simulink model "EEBL_Scenario_01_cs"  (Simulink 7.6)
settings: Solver=ode5  SolverMode=SingleTasking  StartTime=0.0  StopTime=inf  FixedStep=1/100  RelTol=1e-3
PreLoadFcn:
  | check_NUTS_defined;
  | 
  | assignin('base',['model_closed_' bdroot],false);addpath('../includes_V2x');
InitFcn:
  | PreScanExperimentInitFcn(bdroot)
StopFcn:
  | PreScanExperimentStopFcn(bdroot)
undefined symbols (not defined in the file or in its folder): acceleration, actorID, actorType, DiscIntNeverNeededParam, GPS_alt, GPS_lat, GPS_long, intmax, lightBarInUse, messageID, publicVehicleType, rotZ, sireneInUse, trafficLightPriority, turnAdvice, velocity, x_ini_VRML, y_ini_VRML, yawRate, z_ini_VRML
libraries: simulink x58, PreScanSimulinkLibrary x12, simulink_extras x10, PreScanUsefulBlocks x6, simulink_need_slupdate x1
(part 10 of 10)

== system EEBL_Scenario_01_cs/Audi_A8_1/Dynamics_Simple/Chassis/MuxDynState/Transformation_BODY2GLOBAL ==
  Vvector_BODY_[m/s] : Inport
  angles_BODYwrtGLOB_[rad] : Inport  Port=2
  Dot Product : DotProduct  InputSameDT=on  OutDataTypeStr=Inherit: Inherit via internal rule
  Dot Product1 : DotProduct  InputSameDT=on  OutDataTypeStr=Inherit: Inherit via internal rule
  Dot Product2 : DotProduct  InputSameDT=on  OutDataTypeStr=Inherit: Inherit via internal rule
  Fcn10 : Fcn  Expr=cos(u(1))*sin(u(2))*sin(u(3))-sin(u(1))*cos(u(3))
  Fcn11 : Fcn  Expr=cos(u(1))*sin(u(2))*cos(u(3))+sin(u(1))*sin(u(3))
  Fcn12 : Fcn  Expr=sin(u(1))*cos(u(2))
  Fcn13 : Fcn  Expr=sin(u(1))*sin(u(2))*sin(u(3))+cos(u(1))*cos(u(3))
  Fcn14 : Fcn  Expr=sin(u(1))*sin(u(2))*cos(u(3))-cos(u(1))*sin(u(3))
  Fcn15 : Fcn  Expr=-sin(u(2))
  Fcn16 : Fcn  Expr=cos(u(2))*sin(u(3))
  Fcn17 : Fcn  Expr=cos(u(2))*cos(u(3))
  Fcn9 : Fcn  Expr=cos(u(1))*cos(u(2))
  Mux1 : Mux  Inputs=9
  Mux3 : Mux  Inputs=3
  Selector : Selector  InputPortWidth=9  IndexOptions=Index vector (dialog)  Indices=[1 2 3]  OutputSizes=1
  Selector1 : Selector  InputPortWidth=9  IndexOptions=Index vector (dialog)  Indices=[4 5 6]  OutputSizes=1
  Selector2 : Selector  InputPortWidth=9  IndexOptions=Index vector (dialog)  Indices=[7 8 9]  OutputSizes=1
  rot_xyz 2 rot_zyx : Selector  InputPortWidth=3  IndexOptions=Index vector (dialog)  Indices=[3 2 1]  OutputSizes=1
  Vvector_GLOBAL_[m/s] : Outport
  wires:
  Fcn9/1 -> Mux1/1
  Fcn10/1 -> Mux1/2
  Fcn11/1 -> Mux1/3
  Fcn12/1 -> Mux1/4
  Fcn13/1 -> Mux1/5
  Fcn14/1 -> Mux1/6
  Fcn15/1 -> Mux1/7
  Fcn16/1 -> Mux1/8
  Fcn17/1 -> Mux1/9
  Mux1/1 -> Selector/1, Selector1/1, Selector2/1  "RotationMatrix Visu"
  Selector/1 -> Dot Product/2
  Vvector_BODY_[m/s]/1 -> Dot Product2/1, Dot Product1/1, Dot Product/1
  Dot Product/1 -> Mux3/1
  Selector1/1 -> Dot Product1/2
  Selector2/1 -> Dot Product2/2
  Dot Product2/1 -> Mux3/3
  Dot Product1/1 -> Mux3/2
  rot_xyz 2 rot_zyx/1 -> Fcn9/1, Fcn10/1, Fcn11/1, Fcn12/1, Fcn13/1, Fcn14/1, Fcn15/1, Fcn16/1, Fcn17/1
  Mux3/1 -> Vvector_GLOBAL_[m/s]/1
  angles_BODYwrtGLOB_[rad]/1 -> rot_xyz 2 rot_zyx/1

== system EEBL_Scenario_01_cs/Audi_A8_1/Dynamics_Simple/Chassis/RearTyre/AlphaRear ==
  In : Inport
  Abs : Abs
  Compare To Constant : simulink/Logic and Bit Operations/Compare To Constant  SystemSampleTime=-1  relop=>  const=0  LogicOutDataTypeMode=uint8  ZeroCross=off
  Enabled Subsystem : Subsystem  TreatAsAtomicUnit=on
  Selector : Selector  IndexOptions=Index vector (dialog)  Indices=1  OutputSizes=1
  Alpha : Outport
  wires:
  Selector/1 -> Abs/1
  Compare To Constant/1 -> Enabled Subsystem/Enable
  Enabled Subsystem/1(Alpha) -> Alpha/1
  In/1 -> Enabled Subsystem/1(In), Selector/1
  Abs/1 -> Compare To Constant/1

== system EEBL_Scenario_01_cs/Audi_A8_1/Dynamics_Simple/Chassis/RearTyre/Configurable Subsystem ==
  In1 : Inport
  In2 : Inport  Port=2
  Integrator : Integrator  ExternalReset=level
  Out1 : Outport
  wires:
  In1/1 -> Integrator/1
  In2/1 -> Integrator/2
  Integrator/1 -> Out1/1

== system EEBL_Scenario_01_cs/Audi_A8_1/Dynamics_Simple/Chassis/RearTyre/Configurable Subsystem1 ==
  In1 : Inport
  In2 : Inport  Port=2
  Integrator : Integrator  ExternalReset=level  LimitOutput=on  UpperSaturationLimit=1  LowerSaturationLimit=-1
  Out1 : Outport
  wires:
  In1/1 -> Integrator/1
  In2/1 -> Integrator/2
  Integrator/1 -> Out1/1

== system EEBL_Scenario_01_cs/Audi_A8_1/Dynamics_Simple/ShiftLogic/Detect Increase/If V0 higher of the from 2->3 shifting velocity ==
  In1 : Inport
  Action Port : ActionPort  PropagateVarSize=During execution  ActionType=then
  Out1 : Outport
  wires:
  In1/1 -> Out1/1

== system EEBL_Scenario_01_cs/Audi_A8_1/Dynamics_Simple/ShiftLogic/Detect Increase/Other ==
  In1 : Inport
  Action Port : ActionPort  PropagateVarSize=During execution  ActionType=else
  Data Type Conversion : DataTypeConversion  OutDataTypeStr=double
  Detect Increase : simulink/Logic and Bit Operations/Detect Increase  SystemSampleTime=-1  vinit=0.0
  Out1 : Outport
  wires:
  In1/1 -> Detect Increase/1
  Detect Increase/1 -> Data Type Conversion/1
  Data Type Conversion/1 -> Out1/1

== system EEBL_Scenario_01_cs/Audi_A8_1/Dynamics_Simple/Transmission/Transmission_Ratio/If Action Neutral ==
  In1 : Inport
  Action Port : ActionPort  InitializeStates=reset  PropagateVarSize=During execution  ActionType=then
  Out1 : Outport
  wires:
  In1/1 -> Out1/1

== system EEBL_Scenario_01_cs/Audi_A8_1/Dynamics_Simple/Transmission/Transmission_Ratio/If Action Normal ==
  In1 : Inport
  Action Port : ActionPort  InitializeStates=reset  PropagateVarSize=During execution  ActionType=else
  Out1 : Outport
  wires:
  In1/1 -> Out1/1

== system EEBL_Scenario_01_cs/Audi_A8_1/Dynamics_Simple/Transmission/Transmission_Ratio/If Action Reverse ==
  In1 : Inport
  Action Port : ActionPort  InitializeStates=reset  PropagateVarSize=During execution  ActionType=elseif
  Reverse : Gain  Gain=-1
  Out1 : Outport
  wires:
  Reverse/1 -> Out1/1
  In1/1 -> Reverse/1

== system EEBL_Scenario_01_cs/Audi_A8_1/Trajectories/Traj2State1/Traj2State2/MuxState ==
  x [m] : Inport
  y [m] : Inport  Port=2
  z [m] : Inport  Port=3
  dx [m/s] : Inport  Port=4
  dy [m/s] : Inport  Port=5
  dz [m/s] : Inport  Port=6
  R [rad] : Inport  Port=7
  P [rad] : Inport  Port=8
  Y [rad] : Inport  Port=9
  Mux : Mux  Inputs=9
  state : Outport
  wires:
  z [m]/1 -> Mux/3
  y [m]/1 -> Mux/2
  x [m]/1 -> Mux/1
  Y [rad]/1 -> Mux/9
  P [rad]/1 -> Mux/8
  R [rad]/1 -> Mux/7
  dz [m/s]/1 -> Mux/6
  dy [m/s]/1 -> Mux/5
  dx [m/s]/1 -> Mux/4
  Mux/1 -> state/1

== system EEBL_Scenario_01_cs/Audi_A8_1/Trajectories/Traj2State1/Traj2State2/Traj2MuxState_Ext ==
  Traj : Inport
  Terminator{1..9} (9 alike) : Terminator
  demux : Subsystem
  x [m] : Outport
  y [m] : Outport  Port=2
  z [m] : Outport  Port=3
  dx [m/s] : Outport  Port=4
  dy [m/s] : Outport  Port=5
  dz [m/s] : Outport  Port=6
  R [rad] : Outport  Port=7
  P [rad] : Outport  Port=8
  Y [rad] : Outport  Port=9
  wires:
  demux/9(Y) -> Y [rad]/1
  demux/7(R) -> R [rad]/1
  demux/5(vely) -> dy [m/s]/1
  demux/4(velx) -> dx [m/s]/1
  demux/10(velR) -> Terminator4/1
  demux/11(velP) -> Terminator5/1
  demux/12(velY) -> Terminator1/1
  demux/13(accx) -> Terminator8/1
  demux/14(accy) -> Terminator9/1
  demux/15(accz) -> Terminator7/1
  demux/18(accY) -> Terminator2/1
  demux/16(accR) -> Terminator3/1
  demux/17(accP) -> Terminator6/1
  demux/3(z) -> z [m]/1
  Traj/1 -> demux/1(traj)
  demux/6(velz) -> dz [m/s]/1
  demux/1(x) -> x [m]/1
  demux/2(y) -> y [m]/1
  demux/8(P) -> P [rad]/1

== system EEBL_Scenario_01_cs/BMW_X5_1/Trajectories/ElapsedTrack1/MuxState/Substitute 90 & 270 deg (and its plurals) ==
  Angle [rad] : Inport
  270 deg detection : simulink/Model Verification/Check  Static Gap  Description=u <= 269.5 || 270.5 <= u  SystemSampleTime=-1  max=270.5  max_included=on  min=269.5  min_included=on  enabled=on  stopWhenAssertionFail=off  export=on  icon=graphic
  90 deg detection : simulink/Model Verification/Check  Static Gap  Description=u <= 89.5 || 90.5 <= u  SystemSampleTime=-1  max=90.5  max_included=on  min=89.5  min_included=on  enabled=on  stopWhenAssertionFail=off  export=on  icon=graphic
  Angle 0-360 deg limiter : Subsystem
  Degrees to Radians : simulink_extras/Transformations/Degrees to Radians  SystemSampleTime=-1
  Radians to Degrees : simulink_extras/Transformations/Radians to Degrees  SystemSampleTime=-1
  Substitution  Value : Constant  Value=269.5
  Substitution Value : Constant  Value=89.5
  Switch : Switch  Threshold=0.5
  Switch1 : Switch  Threshold=0.5
  Subst Angle [rad] : Outport
  wires:
  Angle [rad]/1 -> Radians to Degrees/1
  Degrees to Radians/1 -> Subst Angle [rad]/1
  Radians to Degrees/1 -> Angle 0-360 deg limiter/1(Angle [deg])
  Switch1/1 -> Degrees to Radians/1
  Substitution  Value/1 -> Switch1/3
  270 deg detection/1 -> Switch1/2
  Switch/1 -> Switch1/1, 270 deg detection/1
  Substitution Value/1 -> Switch/3
  90 deg detection/1 -> Switch/2
  Angle 0-360 deg limiter/1(LimAngle [deg]) -> 90 deg detection/1, Switch/1

== system EEBL_Scenario_01_cs/BMW_X5_1/Trajectories/Traj2State1/Traj2State2/MuxState ==
  x [m] : Inport
  y [m] : Inport  Port=2
  z [m] : Inport  Port=3
  dx [m/s] : Inport  Port=4
  dy [m/s] : Inport  Port=5
  dz [m/s] : Inport  Port=6
  R [rad] : Inport  Port=7
  P [rad] : Inport  Port=8
  Y [rad] : Inport  Port=9
  Mux : Mux  Inputs=9
  state : Outport
  wires:
  z [m]/1 -> Mux/3
  y [m]/1 -> Mux/2
  x [m]/1 -> Mux/1
  Y [rad]/1 -> Mux/9
  P [rad]/1 -> Mux/8
  R [rad]/1 -> Mux/7
  dz [m/s]/1 -> Mux/6
  dy [m/s]/1 -> Mux/5
  dx [m/s]/1 -> Mux/4
  Mux/1 -> state/1

== system EEBL_Scenario_01_cs/BMW_X5_1/Trajectories/Traj2State1/Traj2State2/Traj2MuxState_Ext ==
  Traj : Inport
  Terminator{1..9} (9 alike) : Terminator
  demux : Subsystem
  x [m] : Outport
  y [m] : Outport  Port=2
  z [m] : Outport  Port=3
  dx [m/s] : Outport  Port=4
  dy [m/s] : Outport  Port=5
  dz [m/s] : Outport  Port=6
  R [rad] : Outport  Port=7
  P [rad] : Outport  Port=8
  Y [rad] : Outport  Port=9
  wires:
  demux/9(Y) -> Y [rad]/1
  demux/7(R) -> R [rad]/1
  demux/5(vely) -> dy [m/s]/1
  demux/4(velx) -> dx [m/s]/1
  demux/10(velR) -> Terminator4/1
  demux/11(velP) -> Terminator5/1
  demux/12(velY) -> Terminator1/1
  demux/13(accx) -> Terminator8/1
  demux/14(accy) -> Terminator9/1
  demux/15(accz) -> Terminator7/1
  demux/18(accY) -> Terminator2/1
  demux/16(accR) -> Terminator3/1
  demux/17(accP) -> Terminator6/1
  demux/3(z) -> z [m]/1
  Traj/1 -> demux/1(traj)
  demux/6(velz) -> dz [m/s]/1
  demux/1(x) -> x [m]/1
  demux/2(y) -> y [m]/1
  demux/8(P) -> P [rad]/1

== system EEBL_Scenario_01_cs/BMW_X5_1/vehicle CAM generator/CAM generation/maybe/If Action Subsystem ==
  x [m] : Inport
  y [m] : Inport  Port=2
  z [m] : Inport  Port=3
  rotZ [deg] : Inport  Port=4
  velocity [m/s] : Inport  Port=5
  Action Port : ActionPort  PropagateVarSize=During execution  ActionType=then
  Constant : Constant
  Data Store Write : DataStoreWrite  DataStoreName=CAM_velocity
  Data Store Write1 : DataStoreWrite  DataStoreName=CAM_heading
  Data Store Write2 : DataStoreWrite  DataStoreName=CAM_x
  Data Store Write3 : DataStoreWrite  DataStoreName=CAM_y
  Data Store Write4 : DataStoreWrite  DataStoreName=CAM_z
  Data Store Write5 : DataStoreWrite  DataStoreName=CAM_time
  Digital Clock1 : DigitalClock  SampleTime=0.01
  Out1 : Outport  InitialOutput=0
  wires:
  Constant/1 -> Out1/1
  velocity [m/s]/1 -> Data Store Write/1
  rotZ [deg]/1 -> Data Store Write1/1
  x [m]/1 -> Data Store Write2/1
  y [m]/1 -> Data Store Write3/1
  z [m]/1 -> Data Store Write4/1
  Digital Clock1/1 -> Data Store Write5/1

== system EEBL_Scenario_01_cs/BMW_X5_1/vehicle CAM generator/CAM generation/maybe/If Action Subsystem1 ==
  Action Port : ActionPort  PropagateVarSize=During execution  ActionType=else
  Constant : Constant  Value=0
  Out1 : Outport  InitialOutput=0
  wires:
  Constant/1 -> Out1/1

== system EEBL_Scenario_01_cs/Audi_A8_1/Dynamics_Simple/Chassis/Bicycle_model_[XYZ]/X_Motion/Air&RoadResistance ==
  vx_[ms-1] : Inport
  Gain : Gain  Gain=1/p.Rw
  Road & Aerodyn Resistances : Fcn  Expr=p.Rroad + p.Rair*u^2
  Saturation1 : Saturate  UpperLimit=5/15  LowerLimit=-5/15
  Sign : Signum
  "[ms-1] 2 [rads-1]" : Gain  Gain=1/p.Rw  SaturateOnIntegerOverflow=on  OutDataTypeStr=Inherit: Same as input  ParamDataTypeStr=Inherit: Same as input
  signed load1 : Product  SaturateOnIntegerOverflow=on  InputSameDT=on  OutDataTypeStr=Inherit: Same as first input
  Resistance_Force : Outport
  wires:
  signed load1/1 -> Resistance_Force/1  "F_[N]"
  vx_[ms-1]/1 -> Road & Aerodyn Resistances/1, "[ms-1] 2 [rads-1]"/1
  Saturation1/1 -> Sign/1
  "[ms-1] 2 [rads-1]"/1 -> Saturation1/1
  Road & Aerodyn Resistances/1 -> Gain/1  "ResistanceTorque_[Nm]"
  Sign/1 -> signed load1/2  "sign"
  Gain/1 -> signed load1/1  "Resistance Force_[N]"

== system EEBL_Scenario_01_cs/Audi_A8_1/Dynamics_Simple/Chassis/Bicycle_model_[XYZ]/X_Motion/BrakeSystem ==
  vx_[ms-1] : Inport
  BrakePressure_[bar] : Inport  Port=2
  Gain : Gain  Gain=1/p.Rw
  Saturation : Saturate  UpperLimit=p.PBrakeMax  LowerLimit=0
  Saturation1 : Saturate  UpperLimit=5/15  LowerLimit=-5/15
  Sign : Signum
  "[ms-1] 2 [rads-1]" : Gain  Gain=1/p.Rw  SaturateOnIntegerOverflow=on  OutDataTypeStr=Inherit: Same as input  ParamDataTypeStr=Inherit: Same as input
  braking Q factor : Gain  Gain=p.Qfac  SaturateOnIntegerOverflow=on  OutDataTypeStr=Inherit: Same as input  ParamDataTypeStr=Inherit: Same as input
  signed load1 : Product  SaturateOnIntegerOverflow=on  InputSameDT=on  OutDataTypeStr=Inherit: Same as first input
  BrakeForce : Outport
  BrakeTorqueAbs : Outport  Port=2
  wires:
  braking Q factor/1 -> BrakeTorqueAbs/1, Gain/1
  BrakePressure_[bar]/1 -> Saturation/1
  Saturation/1 -> braking Q factor/1
  vx_[ms-1]/1 -> "[ms-1] 2 [rads-1]"/1
  Saturation1/1 -> Sign/1
  "[ms-1] 2 [rads-1]"/1 -> Saturation1/1
  Sign/1 -> signed load1/2  "sign"
  signed load1/1 -> BrakeForce/1
  Gain/1 -> signed load1/1

== system EEBL_Scenario_01_cs/Audi_A8_1/Dynamics_Simple/Chassis/Bicycle_model_[XYZ]/X_Motion/Configurable Subsystem ==
  In1 : Inport
  In2 : Inport  Port=2
  In3 : Inport  Port=3
  Integrator : Integrator  ExternalReset=level  InitialConditionSource=external
  Out1 : Outport
  wires:
  In1/1 -> Integrator/1
  In2/1 -> Integrator/2
  In3/1 -> Integrator/3
  Integrator/1 -> Out1/1

== system EEBL_Scenario_01_cs/Audi_A8_1/Dynamics_Simple/Chassis/Bicycle_model_[XYZ]/X_Motion/Configurable Subsystem1 ==
  In1 : Inport
  Torsional damping : TransferFcn  Denominator=[0.1 1]
  Out1 : Outport
  wires:
  In1/1 -> Torsional damping/1
  Torsional damping/1 -> Out1/1

== system EEBL_Scenario_01_cs/Audi_A8_1/Dynamics_Simple/Chassis/Bicycle_model_[XYZ]/X_Motion/Max RPM and zero- velocity detection ==
  note: Set to zero after infinite small time-step
  note: Zero velocity detection
  ax : Inport
  Drive Torque : Inport  Port=2
  Brake Torque : Inport  Port=3
  v0 : Inport  Port=4
  vx : Inport  Port=5
  Abs : Abs
  Abs1 : Abs
  Compare To Zero : simulink/Logic and Bit Operations/Compare To Zero  SystemSampleTime=-1  relop=<=  LogicOutDataTypeMode=boolean  ZeroCross=off
  Compare To Zero1 : simulink/Logic and Bit Operations/Compare To Zero  SystemSampleTime=-1  relop=>=  LogicOutDataTypeMode=boolean  ZeroCross=off
  Compare To Zero2 : simulink/Logic and Bit Operations/Compare To Zero  SystemSampleTime=-1  relop=>=  LogicOutDataTypeMode=boolean  ZeroCross=off
  Compare To Zero3 : simulink/Logic and Bit Operations/Compare To Zero  SystemSampleTime=-1  relop=<=  LogicOutDataTypeMode=boolean  ZeroCross=off
  Configurable Subsystem : Subsystem  BlockChoice=Step  mask{ComputationMode=ComputationMode}
      mask prompts: ComputationMode "Compuation mode:"
      mask init:
      | SetComputationMode(gcb,ComputationMode);
      settings: AttributesFormatString=%<BlockChoice>  OpenFcn=BringToFront(gcb);  MemberBlocks=Discrete Step,Step
      settings: TemplateBlock=|
      | PreScanSimulinkLibrary/Configurable Subsystems/Step Function/Configurable
      | Subsystem
  Constant : Constant
  Constant1 : Constant
  Logical Operator : Logic  AllPortsSameDT=off  OutDataTypeStr=boolean
  Logical Operator1 : Logic  AllPortsSameDT=off  OutDataTypeStr=boolean
  Logical Operator2 : Logic  Operator=NOT  AllPortsSameDT=off  OutDataTypeStr=boolean
  Logical Operator3 : Logic  AllPortsSameDT=off  OutDataTypeStr=boolean
  Logical Operator4 : Logic  Operator=OR  AllPortsSameDT=off  OutDataTypeStr=boolean
  Memory : Memory
  Memory1 : Memory
  Memory2 : Memory
  Product : Product  RndMeth=Zero
  Relational Operator : RelationalOperator  Operator=<  OutDataTypeStr=boolean
  SR-Memory : Subsystem
  Sum : Sum  Inputs=|-+
  Switch : Switch  Criteria=u2 ~= 0  Threshold=0.5
  ax is 0 : Constant  Value=0
  ax_out : Outport
  vx_reset : Outport  Port=2
  x0 : Outport  Port=3
  wires:
  Logical Operator4/1 -> Logical Operator1/1
  vx/1 -> Compare To Zero/1, Compare To Zero2/1, Memory2/1, Memory/1  "vx"
  Memory2/1 -> Compare To Zero3/1
  Compare To Zero2/1 -> Logical Operator3/1
  Compare To Zero3/1 -> Logical Operator3/2
  Logical Operator3/1 -> Logical Operator4/2  "zero-crossing backward"
  Memory/1 -> Compare To Zero1/1
  Compare To Zero/1 -> Logical Operator/1
  Compare To Zero1/1 -> Logical Operator/2
  Logical Operator/1 -> Logical Operator4/1  "zero-crossing forward"
  Abs/1 -> Relational Operator/1
  Abs1/1 -> Relational Operator/2
  Drive Torque/1 -> Abs/1
  Brake Torque/1 -> Abs1/1
  Relational Operator/1 -> Logical Operator1/2, Logical Operator2/1
  Logical Operator1/1 -> SR-Memory/2(Set)
  Constant/1 -> SR-Memory/1(Signal)
  Logical Operator2/1 -> SR-Memory/3(Reset)
  SR-Memory/1(Out) -> Sum/1, Memory1/1
  Switch/1 -> ax_out/1
  Sum/1 -> Switch/2
  ax is 0/1 -> Switch/3
  Constant1/1 -> Sum/2
  v0/1 -> Product/1
  Product/1 -> x0/1
  Configurable Subsystem/1(Out1) -> Product/2
  ax/1 -> Switch/1  "ax"
  Memory1/1 -> vx_reset/1  "vx"

== system EEBL_Scenario_01_cs/Audi_A8_1/Dynamics_Simple/Chassis/Bicycle_model_[XYZ]/Y & Yaw_Motion/Configurable Subsystem ==
  In1 : Inport
  In2 : Inport  Port=2
  Integrator : Integrator  ExternalReset=level
  Out1 : Outport
  wires:
  In1/1 -> Integrator/1
  In2/1 -> Integrator/2
  Integrator/1 -> Out1/1

== system EEBL_Scenario_01_cs/Audi_A8_1/Dynamics_Simple/Chassis/Bicycle_model_[XYZ]/Y & Yaw_Motion/Configurable Subsystem1 ==
  In1 : Inport
  Integrator : Integrator
  Out1 : Outport
  wires:
  In1/1 -> Integrator/1
  Integrator/1 -> Out1/1

== system EEBL_Scenario_01_cs/Audi_A8_1/Dynamics_Simple/Chassis/Bicycle_model_[XYZ]/Y & Yaw_Motion/Configurable Subsystem2 ==
  In1 : Inport
  In2 : Inport  Port=2
  Integrator : Integrator  ExternalReset=level
  Out1 : Outport
  wires:
  In1/1 -> Integrator/1
  In2/1 -> Integrator/2
  Integrator/1 -> Out1/1

== system EEBL_Scenario_01_cs/Audi_A8_1/Dynamics_Simple/Chassis/Bicycle_model_[XYZ]/Z, Pitch_Motion & Roll_Motion/Configurable Subsystem ==
  In1 : Inport
  Integrator : Integrator  LimitOutput=on  UpperSaturationLimit=5*pi/180  LowerSaturationLimit=-5*pi/180
  Out1 : Outport
  wires:
  In1/1 -> Integrator/1
  Integrator/1 -> Out1/1

== system EEBL_Scenario_01_cs/Audi_A8_1/Dynamics_Simple/Chassis/Bicycle_model_[XYZ]/Z, Pitch_Motion & Roll_Motion/Configurable Subsystem1 ==
  In1 : Inport
  Integrator : Integrator
  Out1 : Outport
  wires:
  In1/1 -> Integrator/1
  Integrator/1 -> Out1/1

== system EEBL_Scenario_01_cs/Audi_A8_1/Dynamics_Simple/Chassis/Bicycle_model_[XYZ]/Z, Pitch_Motion & Roll_Motion/Configurable Subsystem2 ==
  In1 : Inport
  Integrator : Integrator
  Out1 : Outport
  wires:
  In1/1 -> Integrator/1
  Integrator/1 -> Out1/1

== system EEBL_Scenario_01_cs/Audi_A8_1/Dynamics_Simple/Chassis/Bicycle_model_[XYZ]/Z, Pitch_Motion & Roll_Motion/Configurable Subsystem3 ==
  In1 : Inport
  Integrator : Integrator
  Out1 : Outport
  wires:
  In1/1 -> Integrator/1
  Integrator/1 -> Out1/1

== system EEBL_Scenario_01_cs/Audi_A8_1/Dynamics_Simple/Chassis/Bicycle_model_[XYZ]/Z, Pitch_Motion & Roll_Motion/Configurable Subsystem4 ==
  In1 : Inport
  Integrator : Integrator
  Out1 : Outport
  wires:
  In1/1 -> Integrator/1
  Integrator/1 -> Out1/1

== system EEBL_Scenario_01_cs/Audi_A8_1/Dynamics_Simple/Chassis/Bicycle_model_[XYZ]/Z, Pitch_Motion & Roll_Motion/Configurable Subsystem5 ==
  In1 : Inport
  Integrator : Integrator
  Out1 : Outport
  wires:
  In1/1 -> Integrator/1
  Integrator/1 -> Out1/1

== system EEBL_Scenario_01_cs/Audi_A8_1/Dynamics_Simple/Chassis/Bicycle_model_[XYZ]/Z, Pitch_Motion & Roll_Motion/Configurable Subsystem9 ==
  In1 : Inport
  Derivative : Derivative
  Out1 : Outport
  wires:
  In1/1 -> Derivative/1
  Derivative/1 -> Out1/1

== system EEBL_Scenario_01_cs/Audi_A8_1/Dynamics_Simple/Chassis/FrontTyre/AlphaFront/Enabled Subsystem ==
  In : Inport
  Enable : EnablePort  PropagateVarSize=During execution
  AlphaFront : Fcn  Expr=-atan( (u(2)+u(3)*p.a)/u(1) )
  Alpha : Outport  OutputWhenDisabled=reset  InitialOutput=[0]
  wires:
  AlphaFront/1 -> Alpha/1
  In/1 -> AlphaFront/1

== system EEBL_Scenario_01_cs/Audi_A8_1/Dynamics_Simple/Chassis/RearTyre/AlphaRear/Enabled Subsystem ==
  In : Inport
  Enable : EnablePort  PropagateVarSize=During execution
  AlphaRear : Fcn  Expr=-atan( (u(2)-u(3)*p.b)/u(1) )
  Alpha : Outport  OutputWhenDisabled=reset  InitialOutput=[0]
  wires:
  AlphaRear/1 -> Alpha/1
  In/1 -> AlphaRear/1

== system EEBL_Scenario_01_cs/Audi_A8_1/Trajectories/Traj2State1/Traj2State2/Traj2MuxState_Ext/demux ==
  traj : Inport
  Demux : Demux  Outputs=18
  x : Outport
  y : Outport  Port=2
  z : Outport  Port=3
  velx : Outport  Port=4
  vely : Outport  Port=5
  velz : Outport  Port=6
  R : Outport  Port=7
  P : Outport  Port=8
  Y : Outport  Port=9
  velR : Outport  Port=10
  velP : Outport  Port=11
  velY : Outport  Port=12
  accx : Outport  Port=13
  accy : Outport  Port=14
  accz : Outport  Port=15
  accR : Outport  Port=16
  accP : Outport  Port=17
  accY : Outport  Port=18
  wires:
  Demux/18 -> accY/1
  Demux/17 -> accP/1
  Demux/16 -> accR/1
  Demux/15 -> accz/1
  Demux/14 -> accy/1
  Demux/13 -> accx/1
  Demux/12 -> velY/1
  Demux/11 -> velP/1
  Demux/10 -> velR/1
  Demux/9 -> velz/1
  Demux/8 -> vely/1
  Demux/7 -> velx/1
  Demux/6 -> Y/1
  Demux/5 -> P/1
  traj/1 -> Demux/1
  Demux/4 -> R/1
  Demux/3 -> z/1
  Demux/2 -> y/1
  Demux/1 -> x/1

== system EEBL_Scenario_01_cs/BMW_X5_1/Trajectories/ElapsedTrack1/MuxState/Substitute 90 & 270 deg (and its plurals)/Angle 0-360 deg limiter ==
  Angle [deg] : Inport
  Gain : Gain  Gain=1/360
  Gain1 : Gain  Gain=360
  Rounding Function : Rounding
  Sum : Sum  Inputs=|-+
  LimAngle [deg] : Outport
  wires:
  Gain/1 -> Rounding Function/1
  Rounding Function/1 -> Gain1/1
  Gain1/1 -> Sum/1
  Angle [deg]/1 -> Gain/1, Sum/2
  Sum/1 -> LimAngle [deg]/1

== system EEBL_Scenario_01_cs/BMW_X5_1/Trajectories/Traj2State1/Traj2State2/Traj2MuxState_Ext/demux ==
  traj : Inport
  Demux : Demux  Outputs=18
  x : Outport
  y : Outport  Port=2
  z : Outport  Port=3
  velx : Outport  Port=4
  vely : Outport  Port=5
  velz : Outport  Port=6
  R : Outport  Port=7
  P : Outport  Port=8
  Y : Outport  Port=9
  velR : Outport  Port=10
  velP : Outport  Port=11
  velY : Outport  Port=12
  accx : Outport  Port=13
  accy : Outport  Port=14
  accz : Outport  Port=15
  accR : Outport  Port=16
  accP : Outport  Port=17
  accY : Outport  Port=18
  wires:
  Demux/18 -> accY/1
  Demux/17 -> accP/1
  Demux/16 -> accR/1
  Demux/15 -> accz/1
  Demux/14 -> accy/1
  Demux/13 -> accx/1
  Demux/12 -> velY/1
  Demux/11 -> velP/1
  Demux/10 -> velR/1
  Demux/9 -> velz/1
  Demux/8 -> vely/1
  Demux/7 -> velx/1
  Demux/6 -> Y/1
  Demux/5 -> P/1
  traj/1 -> Demux/1
  Demux/4 -> R/1
  Demux/3 -> z/1
  Demux/2 -> y/1
  Demux/1 -> x/1

== system EEBL_Scenario_01_cs/Audi_A8_1/Dynamics_Simple/Chassis/Bicycle_model_[XYZ]/X_Motion/Max RPM and zero- velocity detection/Configurable Subsystem ==
  Step : Step  Time=0.0001  Before=1  After=0  SampleTime=0
  Out1 : Outport
  wires:
  Step/1 -> Out1/1

== system EEBL_Scenario_01_cs/Audi_A8_1/Dynamics_Simple/Chassis/Bicycle_model_[XYZ]/X_Motion/Max RPM and zero- velocity detection/SR-Memory ==
  Signal : Inport
  Set : Inport  Port=2
  Reset : Inport  Port=3
  Constant : Constant  Value=0
  Detect Rise Positive : simulink/Logic and Bit Operations/Detect Rise Positive  SystemSampleTime=-1  vinit=0
  Detect Rise Positive1 : simulink/Logic and Bit Operations/Detect Rise Positive  SystemSampleTime=-1  vinit=0
  Manual Switch : simulink/Signal Routing/Manual Switch  SystemSampleTime=-1  sw=1  action=0  varsize=off
  Manual Switch1 : simulink/Signal Routing/Manual Switch  SystemSampleTime=-1  sw=1  action=0  varsize=off
  Switch : Switch  Criteria=u2 ~= 0
  Switch1 : Switch  Criteria=u2 ~= 0
  Unit Delay : UnitDelay  SampleTime=-1
  Out : Outport
  wires:
  Constant/1 -> Switch1/1
  Switch/1 -> Switch1/3
  Switch1/1 -> Unit Delay/1, Out/1
  Manual Switch1/1 -> Switch1/2
  Reset/1 -> Manual Switch1/2, Detect Rise Positive1/1
  Detect Rise Positive1/1 -> Manual Switch1/1
  Signal/1 -> Switch/1
  Unit Delay/1 -> Switch/3
  Set/1 -> Detect Rise Positive/1, Manual Switch/2
  Detect Rise Positive/1 -> Manual Switch/1
  Manual Switch/1 -> Switch/2

== stateflow chart Audi_A8_1/EEB/EEBL ==
  state EEBL [parallel]
    settings: executionOrder=1
    state vForward
      (junction 20) -> (junction 16) : {bend = 1;}
      (junction 12) -> (junction 17) [order 2] : {bend = 0;}
      (junction 14) -> (junction 34) [order 1] : [(abs(CAM_Heading[i]-selfHeading)<45 || abs(CAM_Heading[i]-selfHeading)>315) || bend == 1 ]
      (default) -> (junction 12)
      (junction 11) -> (junction 17)
      (junction 16) -> (junction 11)
      (junction 30) -> (junction 26) : {vForward = 0;}
      (junction 28) -> (junction 27) : {vForward = 1;}
      (junction 29) -> (junction 28) [order 1] : [((abs(vAngle-selfHeading)<45 || abs(vAngle-selfHeading)>315) && (abs(vDistance*sin(vAngle*d2r))<5.25)) || bend == 1]
      (junction 29) -> (junction 30) [order 2]
      (junction 31) -> (junction 29)
      (junction 33) -> (junction 30)
      (junction 32) -> (junction 31) [order 1] : [vDistance < 100 && (abs(selfGPSAltitude - CAM_GPSAltitude[i]) < 10)]
      (junction 32) -> (junction 33) [order 2]
      (junction 34) -> (junction 32)
      (junction 14) -> (junction 33) [order 2]
      (junction 19) -> (junction 20) [order 1] : [((abs(L/selfVelocity*selfYawRate + selfHeading - CAM_Heading[i]) < 45) || (abs(L/selfVelocity*selfYawRate + selfHeading - CAM_Heading[i]) > 315)) ]
      (junction 17) -> (junction 14)
      (junction 19) -> (junction 11) [order 2] : {bend = 2;}
      (junction 12) -> (junction 13) [order 1] : [((CAM_YawRate[i] > 2 || CAM_YawRate[i] <-2)  && (selfYawRate > 2 || selfYawRate < -2))]
      (junction 13) -> (junction 19) : {R1 = CAM_Velocity[i]/(CAM_YawRate[i]*d2r);
          | R2 = selfVelocity/(selfYawRate*d2r);
          | alfa = CAM_Heading[i]-selfHeading;
          | L = 2*d2r*180*R2*(alfa/360);}
    state dvBreaking
      (junction 23) -> (junction 21)
      (junction 24) -> (junction 22) : {vBreaking = 1;}
      (junction 22) -> (junction 23)
      (junction 25) -> (junction 23) [order 2]
      (junction 25) -> (junction 24) [order 1] : [ (vForward == 1 && CAM_Acceleration[i] < -brakingWarning)]
      (default) -> (junction 25) : /* Velocity */
    state VehicleAngleandDistance
      state vDistance [parallel]
        settings: executionOrder=2
        (junction 41) -> (junction 40) : {c=2*atan2(sqrt(a), sqrt(1-a));}
        (junction 40) -> (junction 15) : {vDistance = 6371000*c;}
        (default) -> (junction 41) : {a = (sin((CAM_GPSLatitude[i]*d2r-selfGPSLatitude*d2r)/2 ))^2+ cos(selfGPSLatitude*d2r)*cos(CAM_GPSLatitude[i]*d2r)*(sin((CAM_GPSLongitude[i]*d2r-selfGPSLongitude*d2r)/2))^2;}
      state vAngle [parallel]
        settings: executionOrder=1
        (default) -> (junction 18) : {vAngle = (atan2(CAM_GPSLatitude[i]-selfGPSLatitude, CAM_GPSLongitude[i] - selfGPSLongitude))/d2r;}
    state Breaking
      (default) -> (junction 36)
      (junction 36) -> (junction 35) : {Breaking = vBreaking;}
    vForward -> dvBreaking
    VehicleAngleandDistance -> vForward
    (junction 37) -> (junction 39) : {i++;}
    Breaking -> (junction 38)
    (junction 38) -> (junction 39) : {i = 0;
        | vBreaking = 0;
        | vForward = 0;}
    dvBreaking -> (junction 37)
    (junction 39) -> Breaking [order 2]
    (junction 39) -> VehicleAngleandDistance [order 1] : [i < CAM_Size && vBreaking != 1 ]
    (default) -> (junction 39) : {i =0;
        | vForward = 0;}
  note: EEB works with continous signal and checks deceleration of vehicles ahead
  data: a local double; alfa local double; bend local double; c local double; i local double; L local double; vAngle local double; vDistance local double; vForward local double; R1 local double; R2 local double; selfGPSLatitude input double; selfGPSLongitude input double; selfGPSAltitude input double; selfHeading input double; selfVelocity input double; selfYawRate input double; CAM_Velocity input double; CAM_Acceleration input double; CAM_YawRate input double; CAM_GPSLatitude input double; CAM_GPSLongitude input double; CAM_GPSAltitude input double; CAM_Heading input double; CAM_Size input double; d2r constant double =pi()/180; Breaking output double; vBreaking local double; brakingWarning constant double =0.4*9.81

== matlab function Audi_A8_1/EEB/Angle mod ==
  data: u input double; y output double
function y = fcn(u)
%#eml

y = mod(u, 360);

== matlab function Audi_A8_1/EEB/vehicle CAM generator/Signal Matrix create ==
  data: CAM_warning input double; CAM output double; CAM_messageID input double; CAM_vehicleID input double; CAM_vehicleType input double; CAM_publicVehicleType input double; CAM_lightBarInUse input double; CAM_sireneInUse input double; CAM_velocity input double; CAM_acceleration input double; CAM_yawRate input double; CAM_turnAdvice input double; CAM_trafficLightPriority input double; CAM_GPSlat input double; CAM_GPSlong input double; CAM_GPSalt input double; CAM_rotZ input double
function CAM = fcn(CAM_warning, CAM_messageID, CAM_vehicleID, CAM_vehicleType, CAM_publicVehicleType, CAM_lightBarInUse, CAM_sireneInUse, CAM_velocity, CAM_acceleration, CAM_yawRate, CAM_turnAdvice, CAM_trafficLightPriority, CAM_GPSlat, CAM_GPSlong, CAM_GPSalt, CAM_rotZ)
%Signal Matrix creation

CAM = [CAM_warning, CAM_messageID, CAM_vehicleID, CAM_vehicleType, CAM_publicVehicleType, CAM_lightBarInUse, CAM_sireneInUse, CAM_velocity, CAM_acceleration, CAM_yawRate, CAM_turnAdvice, CAM_trafficLightPriority, CAM_GPSlat, CAM_GPSlong, CAM_GPSalt, CAM_rotZ];

== matlab function Audi_A8_1/EEB/vehicle CAM generator/Seperate signals ==
  data: CAM_warning output double; CAM input double; CAM_messageID output double; CAM_vehicleID output double; CAM_vehicleType output double; CAM_publicVehicleType output double; CAM_lightBarInUse output double; CAM_sireneInUse output double; CAM_velocity output double; CAM_acceleration output double; CAM_yawRate output double; CAM_turnAdvice output double; CAM_trafficLightPriority output double; CAM_GPSlat output double; CAM_GPSlong output double; CAM_GPSalt output double; CAM_rotZ output double
function [CAM_warning, CAM_messageID, CAM_vehicleID, CAM_vehicleType, CAM_publicVehicleType, CAM_lightBarInUse, CAM_sireneInUse, CAM_velocity, CAM_acceleration, CAM_yawRate, CAM_turnAdvice, CAM_trafficLightPriority, CAM_GPSlat, CAM_GPSlong, CAM_GPSalt, CAM_rotZ] = fcn(CAM)
%Seperate signals

CAM_warning = CAM(:, 1);
CAM_messageID = CAM(:, 2); 
CAM_vehicleID = CAM(:, 3);
CAM_vehicleType = CAM(:, 4);
CAM_publicVehicleType = CAM(:, 5);
CAM_lightBarInUse = CAM(:, 6);
CAM_sireneInUse = CAM(:, 7);
CAM_velocity = CAM(:, 8);
CAM_acceleration = CAM(:, 9);
CAM_yawRate = CAM(:, 10);
CAM_turnAdvice = CAM(:, 11);
CAM_trafficLightPriority = CAM(:, 12);
CAM_GPSlat = CAM(:, 13);
CAM_GPSlong = CAM(:, 14);
CAM_GPSalt = CAM(:, 15);
CAM_rotZ = CAM(:, 16);

== matlab function Audi_A8_1/EEB/vehicle CAM generator/For Iterator Subsystem/Continuous signal ==
  data: CAM input double; CAM_o output double; CAM_old input double; i input double; NoMM input double; tmp_in input double; tmp_out output double
function [CAM_o, tmp_out] = con(CAM, CAM_old, i, NoMM, tmp_in)
%linearization and number of missed frames control
CAM_o = zeros(1, 16);
tmp_out = tmp_in(i);
if (CAM(i, 3) ~= 0)
    if (mod(tmp_in(i), NoMM+1) == 0)
        CAM_o = CAM (i, :);
    end
    tmp_out = tmp_in(i)+1;
else
    CAM_o = CAM_old(i, :);
end
